simulink model "FH_FSK_final"  (R2021b)
settings: Solver=VariableStepAuto  StartTime=0.0  StopTime=4  RelTol=1e-3
libraries: commfilt2 x8, commchan3 x1, commrandsrc3 x1
settings Model: Creator=Sujay  LastModifiedBy=Sujay

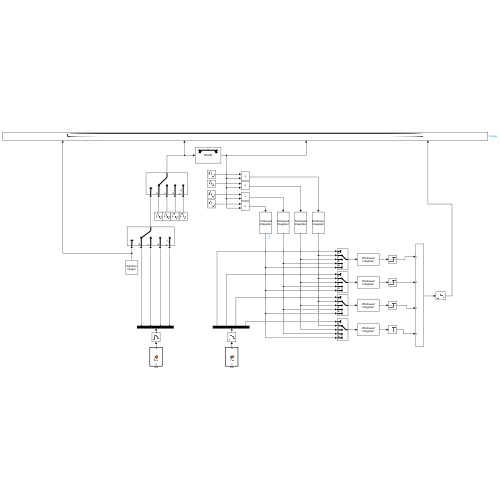
[thumbnail: Simulink's stored preview of the top-level diagram]
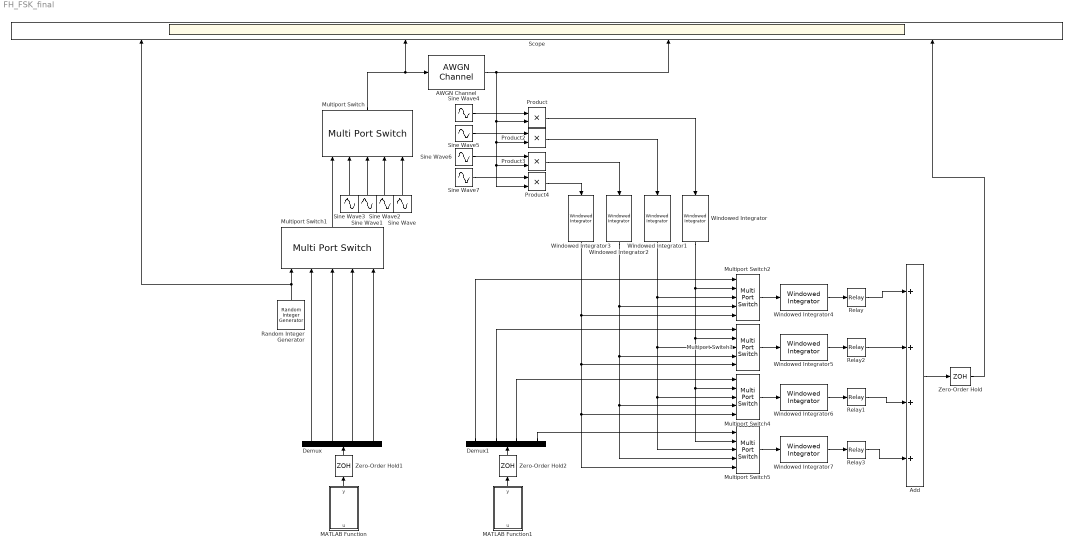
== system FH_FSK_final ==
  AWGN Channel : commchan3/AWGN Channel  InputProcessing=Columns as channels (frame based)  seed=67  noiseMode="Signal to noise ratio  (Eb/No)"  EbNodB=50  EsNodB=10  SNRdB=10  bitsPerSym=1  Ps=1  Tsym=1  variance=1
  Add : Sum  Inputs=++++
  Demux : Demux
  Demux1 : Demux
  MATLAB Function : MATLAB Function  TreatAsAtomicUnit=on
  MATLAB Function1 : MATLAB Function  TreatAsAtomicUnit=on
  Multiport Switch : MultiPortSwitch  DataPortOrder=Specify indices  Inputs=4  DataPortIndices={0, 1, 2, 3}
  Multiport Switch{1..5} (5 alike) : MultiPortSwitch  DataPortOrder=Zero-based contiguous  Inputs=4  zeroidx=on
  Product{,2..4} (4 alike) : Product
  Random Integer Generator : commrandsrc3/Random Integer Generator  SetSize=4  SeedSource=Auto  Seed=0  SampleTime=0.5  SamplesPerFrame=1  OutputDataType=double  SimulateUsing=Interpreted execution
  Relay : Relay  OnSwitchValue=4000  OffSwitchValue=3000  OnOutputValue=0
  Relay1 : Relay  OnSwitchValue=4000  OffSwitchValue=3000  OnOutputValue=2
  Relay2 : Relay  OnSwitchValue=4000  OffSwitchValue=3000
  Relay3 : Relay  OnSwitchValue=4000  OffSwitchValue=3000  OnOutputValue=3
  Scope : Scope  NumInputPorts=4
  Sine Wave : Sin  Frequency=2 * pi * 40  SampleTime=0.001
  Sine Wave1 : Sin  Frequency=2 * pi * 20  SampleTime=0.001
  Sine Wave2 : Sin  Frequency=2 * pi * 30  SampleTime=0.001
  Sine Wave3 : Sin  Frequency=2 * pi * 10  SampleTime=0.001
  Sine Wave4 : Sin  Frequency=2 * pi * 10  SampleTime=0.001
  Sine Wave5 : Sin  Frequency=2 * pi * 20  SampleTime=0.001
  Sine Wave6 : Sin  Frequency=2 * pi * 30  SampleTime=0.001
  Sine Wave7 : Sin  Frequency=2 * pi * 40  SampleTime=0.001
  Windowed Integrator{,1..7} (8 alike) : commfilt2/Windowed Integrator  integperiod=100  InputProcessing=Columns as channels (frame based)  roundingMode=Floor  overflowMode=off  coeffDataTypeStr=Inherit: Same word length as input  coeffMin=[]  coeffMax=[]  coeffLastDataTypeStr=Inherit: Same word length as input  accumDataTypeStr=Inherit: Same as product output  accumLastDataTypeStr=Inherit: Same as product output  outputDataTypeStr=Inherit: Same as accumulator  outputMin=[]  outputMax=[]  outputLastDataTypeStr=Inherit: Same as accumulator
      settings: SourceProductBaseCode=CM
  Zero-Order Hold : ZeroOrderHold  SampleTime=0.5
  Zero-Order Hold1 : ZeroOrderHold  SampleTime=0.5
  Zero-Order Hold2 : ZeroOrderHold  SampleTime=0.5
  wires:
  Sine Wave/1 -> Multiport Switch/5
  Sine Wave2/1 -> Multiport Switch/4
  Sine Wave1/1 -> Multiport Switch/3
  Sine Wave3/1 -> Multiport Switch/2
  Multiport Switch/1 -> AWGN Channel/1, Scope/2
  Sine Wave4/1 -> Product/1
  Sine Wave5/1 -> Product2/1
  Sine Wave6/1 -> Product3/1
  Sine Wave7/1 -> Product4/1
  AWGN Channel/1 -> Scope/3, Product/2, Product2/2, Product3/2, Product4/2
  Product/1 -> Windowed Integrator/1
  Product4/1 -> Windowed Integrator3/1
  Product3/1 -> Windowed Integrator2/1
  Product2/1 -> Windowed Integrator1/1
  Relay/1 -> Add/1
  Relay1/1 -> Add/3
  Relay2/1 -> Add/2
  Relay3/1 -> Add/4
  Add/1 -> Zero-Order Hold/1
  Random Integer Generator/1 -> Scope/1, Multiport Switch1/1
  Multiport Switch1/1 -> Multiport Switch/1
  Windowed Integrator3/1 -> Multiport Switch5/5, Multiport Switch4/5, Multiport Switch3/5, Multiport Switch2/5
  Windowed Integrator2/1 -> Multiport Switch5/4, Multiport Switch4/4, Multiport Switch3/4, Multiport Switch2/4
  Windowed Integrator1/1 -> Multiport Switch5/3, Multiport Switch4/3, Multiport Switch3/3, Multiport Switch2/3
  Windowed Integrator/1 -> Multiport Switch5/2, Multiport Switch4/2, Multiport Switch3/2, Multiport Switch2/2
  Multiport Switch2/1 -> Windowed Integrator4/1
  Multiport Switch3/1 -> Windowed Integrator5/1
  Multiport Switch4/1 -> Windowed Integrator6/1
  Multiport Switch5/1 -> Windowed Integrator7/1
  Demux/1 -> Multiport Switch1/2
  Demux/4 -> Multiport Switch1/5
  Demux/3 -> Multiport Switch1/4
  Demux/2 -> Multiport Switch1/3
  Zero-Order Hold1/1 -> Demux/1
  Windowed Integrator4/1 -> Relay/1
  Windowed Integrator7/1 -> Relay3/1
  Windowed Integrator6/1 -> Relay1/1
  Windowed Integrator5/1 -> Relay2/1
  MATLAB Function/1(y) -> Zero-Order Hold1/1
  Zero-Order Hold/1 -> Scope/4
  Demux1/2 -> Multiport Switch3/1
  Demux1/3 -> Multiport Switch4/1
  Zero-Order Hold2/1 -> Demux1/1
  Demux1/4 -> Multiport Switch5/1
  Demux1/1 -> Multiport Switch2/1
  MATLAB Function1/1(y) -> Zero-Order Hold2/1

== matlab function FH_FSK_final/MATLAB Function ==
  data: y output; u input
function y = fcn(u)

rng(5)
y = randperm(4)' - 1;

== matlab function FH_FSK_final/MATLAB Function1 ==
  data: y output; u input
function y = fcn(u)

rng(5)
y = randperm(4)' - 1;
